simulink library "Sky_Temperature"  (Simulink 8.2)
settings: Solver=ode45  StartTime=0.0  StopTime=10.0  RelTol=1e-3
settings Model: Creator=drhf  LastModifiedBy=drhf

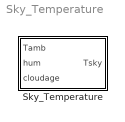
== system Sky_Temperature ==
  Sky_Temperature : Subsystem  mask(Sky Temperature){tskymodel=on}
      mask prompts: tskymodel "Include time correction (cos-term in Berdahl equation)"
      mask help:
      | Calculates the skytemperature. If humidity data is availabe, the model of Berdahl and Martin 1984 for low clouds (1000 m) is used.
      | Without humidity data, the model of Unsworth with corrected parameters of Feist 1994 is chosen.
      | INPUT VECTOR:
      |   tamb : ambient temperature [°C]
      |   hum  : humidity [%]
      |   cloud: index of cloudness [0,1]
      |
      | OUTPUT VECTOR:
      |   tsky : sky temperature [°C]
      |
      | The calculation can also be used in m-files with the skytemperature.m function.
      mask Help: web(fullfile(path_carnot('help'),'Sky_Temperature.html'),'-helpbrowser')

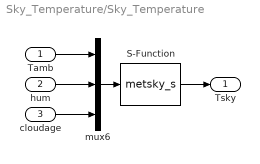
== system Sky_Temperature/Sky_Temperature ==
  Tamb : Inport
  hum : Inport  Port=2
  cloudage : Inport  Port=3
  S-Function : S-Function  FunctionName=metsky_s  Parameters=tskymodel  EnableBusSupport=off
  mux6 : Mux  Inputs=3
  Tsky : Outport
  wires:
  cloudage/1 -> mux6/3
  hum/1 -> mux6/2
  Tamb/1 -> mux6/1
  mux6/1 -> S-Function/1
  S-Function/1 -> Tsky/1
